simulink model "GalvoTransferFuncGetSS"  (R2013a)
settings: Solver=ode45  StartTime=0.0  StopTime=init.StopTime  MinStep=init.MinStepSize  RelTol=1e-3
model workspace: external: MAT-File /home/mainster/CODES_local/matlab_workspace/paramPID1.mat (data not in the file)
values from neighbouring files (symbols this model uses):
  init = struct('TsSens',   30e-6,              'TsSens2',  555e-6,              'TsCtrl',   100e-6,              'StopTime', 50e-3,              'MinStepSize',  10e-6)    [GalvoTransferFuncFeedback_processing_back.m]    (also in GalvoTransferFuncGetSS_processing.m = struct('TsSens',   30e-6,              'TsSens2',  30e-6,   ; Galvo_process_analyze.m = 0)
  PID = sym2tf(eval(pid))    [GalvoModel_v4_sys.m]    (also in GalvoTransferFuncGetSS_processing.m = struct( 'P',    0.392064644185526,              'I',    2068)
undefined symbols (not defined in the file or in its folder): DiscIntNeverNeededParam
libraries: simulink x3
settings Model: Creator=mainster  LastModifiedBy=mainster
settings DebuggingCC: SolverPrmCheckMsg=none

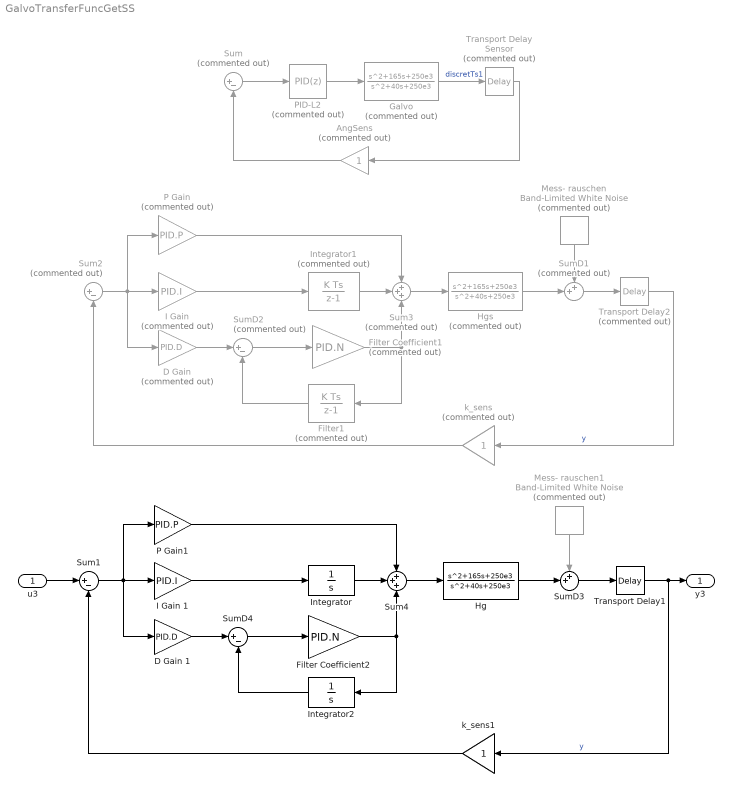
== system GalvoTransferFuncGetSS ==
  u3 : Inport
  AngSens : Gain  Commented=on  SampleTime=init.TsSens
  "D Gain " : Gain  Commented=on  DisableCoverage=on  Gain=PID.D  OutDataTypeStr=Inherit: Inherit via back propagation  SampleTime=PID.Ts
  D Gain 1 : Gain  DisableCoverage=on  Gain=PID.D  OutDataTypeStr=Inherit: Inherit via back propagation
  Filter Coefficient1 : Gain  Commented=on  Gain=PID.N  OutDataTypeStr=Inherit: Inherit via back propagation  SampleTime=PID.Ts
  Filter Coefficient2 : Gain  Gain=PID.N  OutDataTypeStr=Inherit: Inherit via back propagation
  Filter1 : DiscreteIntegrator  Commented=on  DisableCoverage=on  InitialConditionMode=State only (most efficient)  SampleTime=PID.Ts  OutDataTypeStr=Inherit: Inherit via back propagation  ICPrevOutput=DiscIntNeverNeededParam  ICPrevScaledInput=DiscIntNeverNeededParam
  Galvo : TransferFcn  Commented=on  Numerator=[1 165 250e3]  Denominator=[1 40 250e3]
  Hg : TransferFcn  Numerator=[1 165 250e3]  Denominator=[1 40 250e3]
  Hgs : TransferFcn  Commented=on  Numerator=[1 165 250e3]  Denominator=[1 40 250e3]
  "I Gain " : Gain  Commented=on  DisableCoverage=on  Gain=PID.I  OutDataTypeStr=Inherit: Inherit via back propagation  SampleTime=PID.Ts
  I Gain 1 : Gain  DisableCoverage=on  Gain=PID.I  OutDataTypeStr=Inherit: Inherit via back propagation
  Integrator : Integrator
  Integrator1 : DiscreteIntegrator  Commented=on  InitialConditionMode=State only (most efficient)  SampleTime=PID.Ts  OutDataTypeStr=Inherit: Inherit via back propagation  ICPrevOutput=DiscIntNeverNeededParam  ICPrevScaledInput=DiscIntNeverNeededParam
  Integrator2 : Integrator
  Mess- rauschen : simulink/Sources/Band-Limited White Noise  Commented=on  Cov=[0.1e-15]  Ts=0  seed=[23341]
  Mess- rauschen1 : simulink/Sources/Band-Limited White Noise  Commented=on  Cov=[0.1e-15]  Ts=0  seed=[23341]
  P Gain : Gain  Commented=on  Gain=PID.P  SampleTime=PID.Ts
  P Gain1 : Gain  Gain=PID.P
  PID-L2 : simulink/Continuous/PID Controller  Commented=on  Controller=PID  TimeDomain=Discrete-time  SampleTime=PID.Ts  IntegratorMethod=Forward Euler  FilterMethod=Forward Euler  Form=Parallel  P=0.384349742528594  I=2468.66636470386  D=0  N=100  InitialConditionSource=internal  InitialConditionForIntegrator=0  InitialConditionForFilter=0  ExternalReset=none  LimitOutput=off  UpperSaturationLimit=inf  LowerSaturationLimit=-inf  LinearizeAsGain=off  AntiWindupMode=none  Kb=1  TrackingMode=off  Kt=1  PParamMin=[]  PParamMax=[]  IParamMin=[]  IParamMax=[]  DParamMin=[]  DParamMax=[]  NParamMin=[]  NParamMax=[]  KbParamMin=[]  KbParamMax=[]  KtParamMin=[]  KtParamMax=[]  POutMin=[]  POutMax=[]  IOutMin=[]  IOutMax=[]  DOutMin=[]  DOutMax=[]  NOutMin=[]  NOutMax=[]  KbOutMin=[]  KbOutMax=[]  KtOutMin=[]  KtOutMax=[]  IntegratorOutMin=[]  IntegratorOutMax=[]  FilterOutMin=[]  FilterOutMax=[]  SumOutMin=[]  SumOutMax=[]  SumI1OutMin=[]  SumI1OutMax=[]  SumI2OutMin=[]  SumI2OutMax=[]  SumI3OutMin=[]  SumI3OutMax=[]  SumDOutMin=[]  SumDOutMax=[]  SaturationOutMin=[]  SaturationOutMax=[]  IntegratorContinuousStateAttributes=''  IntegratorStateMustResolveToSignalObject=off  IntegratorRTWStateStorageClass=Auto  FilterContinuousStateAttributes=''  FilterStateMustResolveToSignalObject=off  FilterRTWStateStorageClass=Auto
  Sum : Sum  Commented=on  Inputs=|+-  SampleTime=init.TsSens
  Sum1 : Sum  Inputs=|+-
  Sum2 : Sum  Commented=on  Inputs=|+-  SampleTime=init.TsSens
  Sum3 : Sum  Commented=on  Inputs=+++  OutDataTypeStr=Inherit: Inherit via back propagation  SampleTime=PID.Ts
  Sum4 : Sum  Inputs=+++  OutDataTypeStr=Inherit: Inherit via back propagation
  SumD1 : Sum  Commented=on  DisableCoverage=on  Inputs=++|
  SumD2 : Sum  Commented=on  DisableCoverage=on  Inputs=|+-  SampleTime=PID.Ts
  SumD3 : Sum  DisableCoverage=on  Inputs=++|
  SumD4 : Sum  DisableCoverage=on  Inputs=|+-
  Transport Delay Sensor : TransportDelay  Commented=on  DelayTime=init.DelayTime
  Transport Delay1 : TransportDelay  DelayTime=init.DelayTime
  Transport Delay2 : TransportDelay  Commented=on  DelayTime=init.DelayTime
  k_sens : Gain  Commented=on  SampleTime=init.TsSens
  k_sens1 : Gain
  y3 : Outport
  wires:
  Sum/1 -> PID-L2/1
  Galvo/1 -> Transport Delay Sensor/1  "discretTs1"
  PID-L2/1 -> Galvo/1
  AngSens/1 -> Sum/2
  Transport Delay Sensor/1 -> AngSens/1
  Transport Delay2/1 -> k_sens/1  "y"
  k_sens/1 -> Sum2/2
  Hgs/1 -> SumD1/2
  SumD1/1 -> Transport Delay2/1
  Mess- rauschen/1 -> SumD1/1
  "I Gain "/1 -> Integrator1/1
  "D Gain "/1 -> SumD2/1
  SumD2/1 -> Filter Coefficient1/1
  Filter Coefficient1/1 -> Sum3/3, Filter1/1
  Filter1/1 -> SumD2/2
  Integrator1/1 -> Sum3/2
  P Gain/1 -> Sum3/1
  Sum3/1 -> Hgs/1
  Sum2/1 -> P Gain/1, "I Gain "/1, "D Gain "/1
  Transport Delay1/1 -> y3/1, k_sens1/1  "y"
  k_sens1/1 -> Sum1/2
  Hg/1 -> SumD3/2
  SumD3/1 -> Transport Delay1/1
  Mess- rauschen1/1 -> SumD3/1
  I Gain 1/1 -> Integrator/1
  D Gain 1/1 -> SumD4/1
  SumD4/1 -> Filter Coefficient2/1
  Filter Coefficient2/1 -> Integrator2/1, Sum4/3
  Integrator2/1 -> SumD4/2
  P Gain1/1 -> Sum4/1
  Sum4/1 -> Hg/1
  Sum1/1 -> P Gain1/1, I Gain 1/1, D Gain 1/1
  u3/1 -> Sum1/1
  Integrator/1 -> Sum4/2
